simulink model "BLDC_180deg_realVSI"  (R2024a)
settings: Solver=ode15s  StartTime=0.0  StopTime=2  RelTol=1e-3
values from neighbouring files (symbols this model uses):
  D_m = 1e-3    (= 0.001)    [BLDC_Parameters.m]
  J_t = 1e-3    (= 0.001)    [BLDC_Parameters.m]
  L_ss = tau_s * r_s    (= 0.0003657)    [BLDC_Parameters.m]
  lambda_m = torque_const/(3*P/4)    (= 0.00985)    [BLDC_Parameters.m]
  P = 8    [BLDC_Parameters.m]
  r_s = r_pp/2    (= 0.345)    [BLDC_Parameters.m]
  R_vs = 1e6    (= 1000000)    [BLDC_Parameters.m]
  tau_s = 1.06e-3    (= 0.00106)    [BLDC_Parameters.m]
  V_bus = 12    [BLDC_Parameters.m]
libraries: simulink x7, spsMosfetLib x6, spsSeriesRLCBranchLib x4, spsVoltageMeasurementLib x3, spsControlledCurrentSourceLib x3, dspswit3 x1, slpidlib x1, spsPWMGeneratorDCDCLib x1, spsDCVoltageSourceLib x1, sps_lib x1
settings Model: Creator=matthewhasman  LastModifiedBy=matthewhasman

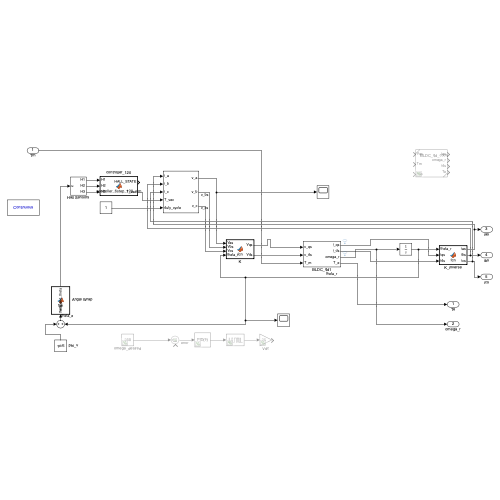
[thumbnail: Simulink's stored preview of the top-level diagram]
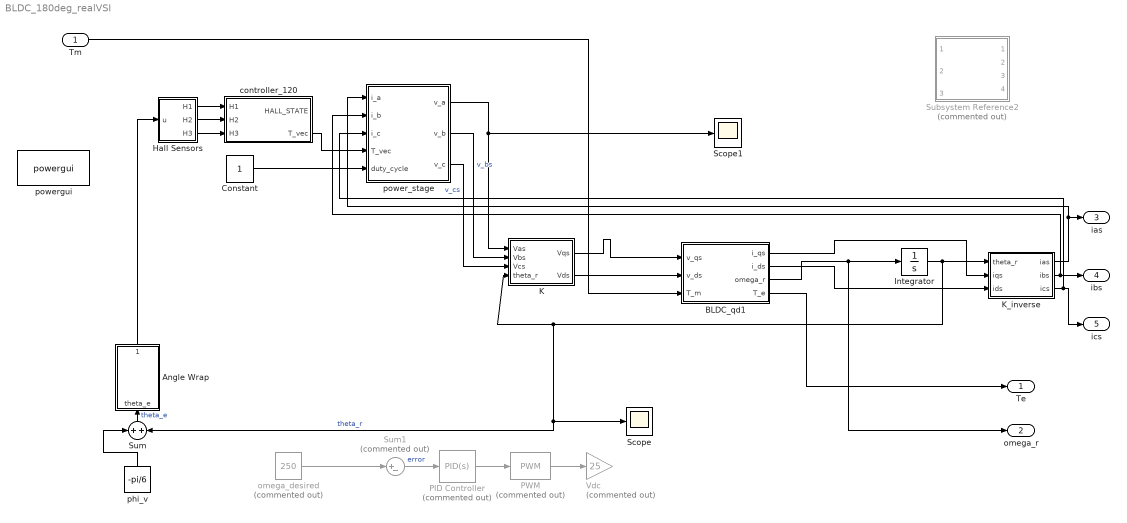
== system BLDC_180deg_realVSI ==
  Tm : Inport
  Angle Wrap : MATLAB Function  TreatAsAtomicUnit=on
  BLDC_qd1 : Subsystem
  Constant : Constant
  Hall Sensors : Subsystem
  Integrator : Integrator
  K : MATLAB Function  TreatAsAtomicUnit=on
  K_inverse : MATLAB Function  TreatAsAtomicUnit=on
  PID Controller : slpidlib/PID Controller  Commented=on  Controller=PID  Form=Parallel  TimeDomain=Continuous-time  UseExternalTs=off  SampleTime=-1  IntegratorMethod=Forward Euler  FilterMethod=Forward Euler  ControllerParametersSource=internal  P=8  I=5  UseKiTs=off  D=1  UseExternalDerivativeSource=off  N=100  UseFilter=on  TunerSelectOption=Transfer Function Based (PID Tuner App)  InitialConditionSource=internal  InitialConditionForIntegrator=0  InitialConditionForFilter=0  DifferentiatorICPrevScaledInput=0  ExternalReset=none  TrackingMode=off  Kt=1  LimitOutput=off  SatLimitsSource=internal  UpperSaturationLimit=inf  LowerSaturationLimit=-inf  LinearizeAsGain=on  AntiWindupMode=none  Kb=1  LimitIntegrator=off  UpperIntegratorSaturationLimit=inf  LowerIntegratorSaturationLimit=-inf  POutMin=[]  POutMax=[]  IOutMin=[]  IOutMax=[]  DOutMin=[]  DOutMax=[]  NOutMin=[]  NOutMax=[]  SumOutMin=[]  SumOutMax=[]  SaturationOutMin=[]  SaturationOutMax=[]  PParamMin=[]  PParamMax=[]  IParamMin=[]  IParamMax=[]  DParamMin=[]  DParamMax=[]  NParamMin=[]  NParamMax=[]  KbParamMin=[]  KbParamMax=[]  KtParamMin=[]  KtParamMax=[]  KbOutMin=[]  KbOutMax=[]  KtOutMin=[]  KtOutMax=[]  IntegratorOutMin=[]  IntegratorOutMax=[]  FilterOutMin=[]  FilterOutMax=[]  SumI1OutMin=[]  SumI1OutMax=[]  SumI2OutMin=[]  SumI2OutMax=[]  SumI3OutMin=[]  SumI3OutMax=[]  SumI4OutMin=[]  SumI4OutMax=[]  SumDOutMin=[]  SumDOutMax=[]  DifferentiatorOutMin=[]  DifferentiatorOutMax=[]  FilterDiffOutCoefMin=[]  FilterDiffOutCoefMax=[]  ReciprocalOutMin=[]  ReciprocalOutMax=[]  SumDenOutMin=[]  SumDenOutMax=[]  SumNumOutMin=[]  SumNumOutMax=[]  DivideOutMin=[]  DivideOutMax=[]  UdiffTsProdOutMin=[]  UdiffTsProdOutMax=[]  NTsProdOutMin=[]  NTsProdOutMax=[]  UintegralTsProdOutMin=[]  UintegralTsProdOutMax=[]  UngainTsProdOutMin=[]  UngainTsProdOutMax=[]  ClampingZeroOutDataTypeStr=Inherit: Inherit via back propagation  ClampingZeroOutMin=[]  ClampingZeroOutMax=[]  FilterDenConstantOutDataTypeStr=Inherit: Inherit via back propagation  FilterDenConstantOutMin=[]  FilterDenConstantOutMax=[]  PCopyOutDataTypeStr=Inherit: Inherit via back propagation  PCopyOutMin=[]  PCopyOutMax=[]  NCopyOutDataTypeStr=Inherit: Inherit via back propagation  NCopyOutMin=[]  NCopyOutMax=[]  IntegratorContinuousStateAttributes=''  IntegratorStateMustResolveToSignalObject=off  IntegratorRTWStateStorageClass=Auto  FilterContinuousStateAttributes=''  FilterStateMustResolveToSignalObject=off  FilterRTWStateStorageClass=Auto  ParallelPVariant=InternalParameters  IdealPVariant=Disabled  IVariant=InternalParameters  DVariant=InternalParameters  IntegratorVariant=Continuous  SatVariant=Disabled  AWVariant=Passthrough  PCopyVariant=Disabled  TRVariant=Disabled  FdbkBlocksVariant=Forward  IdealPFdbkVariant=Disabled  SatFdbkVariant=Disabled  DerivativeFilterVariant=ContFilter  NVariant=InternalParameters  NCopyVariant=Disabled  FilterICVariant=InternalICsFilter  IntegratorICVariant=InternalICs  ExternalResetVariant=Disabled  TRSumVariant=Passthrough  SumFdbkVariant=Disabled  SumVariant=Sum_PID  TsampFilterVariant=InternalTs  TsampNgainVariant=Passthrough  TsampIntegralVariant=Disabled_SignalSpec  ExternalSaturationOutDataTypeStr=Inherit: Same as second input  DerivativeSourceVariant=ErrorSignal
  PWM : simulink/Discontinuities/PWM  Commented=on  DisableCoverage=on  Period=0.0001  InitialDelay=0  DisallowZeroDutyCycle=off  RunAtFixedTimeIntervals=off  SampleTime=0.1
  Scope : Scope
  Scope1 : Scope
  Subsystem Reference2 : Subsystem  Commented=on  ReferencedSubsystem=BLDC_qd_coords
  Sum : Sum
  Sum1 : Sum  Commented=on  Inputs=|+-
  Vdc : Gain  Commented=on  Gain=25
  controller_120 : MATLAB Function  TreatAsAtomicUnit=on
  omega_desired : Constant  Commented=on  Value=250
  phi_v : Constant  Value=-pi/6
  power_stage : Subsystem
  powergui : sps_lib/powergui  Priority=1  SimulationMode=Continuous  SampleTime=50e-6  frequency=60  Iterations=50  frequencyindice=0  Pbase=100e6  ErrMax=1e-4  UnitsV=kV  UnitsW=MW  buscounter=0  FunctionMessages=off  echomessages=off  EnableUseOfTLC=off  CurrentSourceSwitches=off  DisableSnubberDevices=off  DisableRonSwitches=off  DisableVfSwitches=off  DisplayEquations=off  AutomaticDiscreteSolvers=off  SolverType=Tustin/Backward Euler (TBE)  Interpol=off  ExternalGateDelay=off  methode=off  Ts=100  x0status=blocks  SPID=on  SwTol=0  HookPort=off  NonlinearTolerance=1e-4  nMaxIteration=100  ContinueOnMaxIteration=off  RestoreLinks=warning  ResistiveCurrentMeasurement=off  Frange=[0:2:500]  Ylog=off  Xlog=on  ShowGrid=off  save=off  variable=ZData  structure=0  ZoomFFT=off  StartTime=0.0  cycles=1  DisplayStyle=1  fundamental=60  FreqAxis=off  MaxFrequency=1000  frequencyindicesteady=1  RmsSteady=1  display=off
  Te : Outport
  omega_r : Outport  Port=2
  ias : Outport  Port=3
  ibs : Outport  Port=4
  ics : Outport  Port=5
  wires:
  Integrator/1 -> K_inverse/1(theta_r), Scope/1, Sum/2, K/4(theta_r)  "theta_r"
  K/1(Vqs) -> BLDC_qd1/1(v_qs)
  phi_v/1 -> Sum/1
  power_stage/1(v_a) -> Scope1/1, K/1(Vas)
  omega_desired/1 -> Sum1/1
  Sum1/1 -> PID Controller/1  "error"
  PID Controller/1 -> PWM/1
  PWM/1 -> Vdc/1
  Sum/1 -> Angle Wrap/1(theta_e)  "theta_e"
  K_inverse/1(ias) -> power_stage/1(i_a), ias/1
  K_inverse/2(ibs) -> ibs/1, power_stage/2(i_b)
  K_inverse/3(ics) -> power_stage/3(i_c), ics/1
  Angle Wrap/1(wrapped_theta) -> Hall Sensors/1(u)
  power_stage/2(v_b) -> K/2(Vbs)  "v_bs"
  power_stage/3(v_c) -> K/3(Vcs)  "v_cs"
  Hall Sensors/3(H3) -> controller_120/3(H3)
  Hall Sensors/1(H1) -> controller_120/1(H1)
  Hall Sensors/2(H2) -> controller_120/2(H2)
  controller_120/2(T_vec) -> power_stage/4(T_vec)
  Constant/1 -> power_stage/5(duty_cycle)
  K/2(Vds) -> BLDC_qd1/2(v_ds)
  Tm/1 -> BLDC_qd1/3(T_m)
  BLDC_qd1/1(i_qs) -> K_inverse/2(iqs)
  BLDC_qd1/2(i_ds) -> K_inverse/3(ids)
  BLDC_qd1/3(omega_r) -> omega_r/1, Integrator/1
  BLDC_qd1/4(T_e) -> Te/1

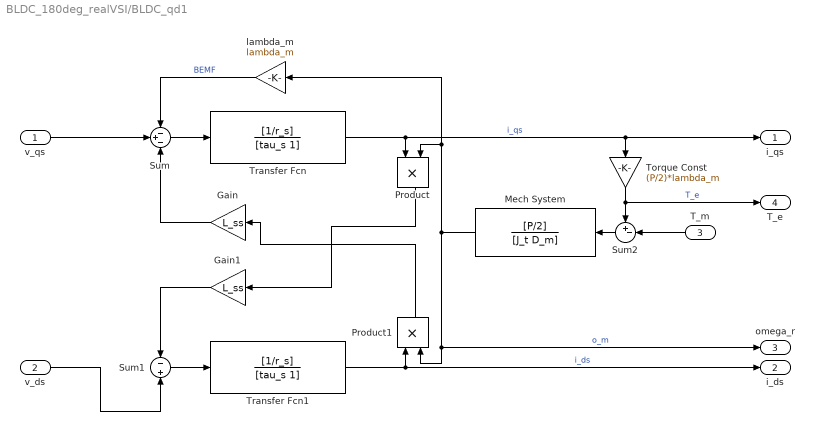
== system BLDC_180deg_realVSI/BLDC_qd1 ==
  v_qs : Inport
  v_ds : Inport  Port=2
  T_m : Inport  Port=3
  Gain : Gain  Gain=L_ss
  Gain1 : Gain  Gain=L_ss
  Mech System : TransferFcn  Numerator=[P/2]  Denominator=[J_t D_m]
  Product : Product
  Product1 : Product
  Sum : Sum  Inputs=-+-
  Sum1 : Sum  Inputs=-+
  Sum2 : Sum  Inputs=+-|
  Torque Const : Gain  Gain=(P/2)*lambda_m
  Transfer Fcn : TransferFcn  Numerator=[1/r_s]  Denominator=[tau_s 1]
  Transfer Fcn1 : TransferFcn  Numerator=[1/r_s]  Denominator=[tau_s 1]
  lambda_m : Gain  Gain=lambda_m
  i_qs : Outport
  i_ds : Outport  Port=2
  omega_r : Outport  Port=3
  T_e : Outport  Port=4
  wires:
  T_m/1 -> Sum2/2
  Sum1/1 -> Transfer Fcn1/1
  Gain1/1 -> Sum1/1
  Product1/1 -> Gain/1
  Transfer Fcn1/1 -> i_ds/1, Product1/1  "i_ds"
  Mech System/1 -> lambda_m/1, Product/2, omega_r/1, Product1/2  "o_m"
  Torque Const/1 -> T_e/1, Sum2/1  "T_e"
  v_ds/1 -> Sum1/2
  Transfer Fcn/1 -> i_qs/1, Torque Const/1, Product/1  "i_qs"
  Product/1 -> Gain1/1
  Gain/1 -> Sum/3
  v_qs/1 -> Sum/2
  Sum/1 -> Transfer Fcn/1
  Sum2/1 -> Mech System/1
  lambda_m/1 -> Sum/1  "BEMF"

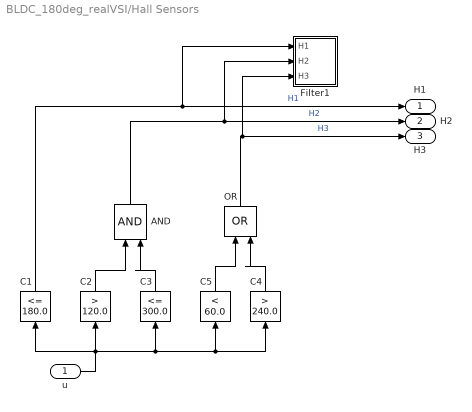
== system BLDC_180deg_realVSI/Hall Sensors ==
  u : Inport
  AND : Logic  IconShape=distinctive  AllPortsSameDT=off  OutDataTypeStr=boolean
  C1 : simulink/Logic and Bit Operations/Compare To Constant  relop=<=  const=180.0  OutDataTypeStr=boolean
  C2 : simulink/Logic and Bit Operations/Compare To Constant  relop=>  const=120.0  OutDataTypeStr=boolean
  C3 : simulink/Logic and Bit Operations/Compare To Constant  relop=<=  const=300.0  OutDataTypeStr=boolean
  C4 : simulink/Logic and Bit Operations/Compare To Constant  relop=>  const=240.0  OutDataTypeStr=boolean
  C5 : simulink/Logic and Bit Operations/Compare To Constant  relop=<  const=60.0  OutDataTypeStr=boolean
  Filter1 : Subsystem
  OR : Logic  Operator=OR  IconShape=distinctive  AllPortsSameDT=off  OutDataTypeStr=boolean
  H1 : Outport
  H2 : Outport  Port=2
  H3 : Outport  Port=3
  wires:
  C4/1 -> OR/2
  C1/1 -> H1/1, Filter1/1(H1)  "H1"
  OR/1 -> H3/1, Filter1/3(H3)  "H3"
  C3/1 -> AND/2
  AND/1 -> H2/1, Filter1/2(H2)  "H2"
  u/1 -> C2/1, C5/1, C4/1, C3/1, C1/1
  C2/1 -> AND/1
  C5/1 -> OR/1

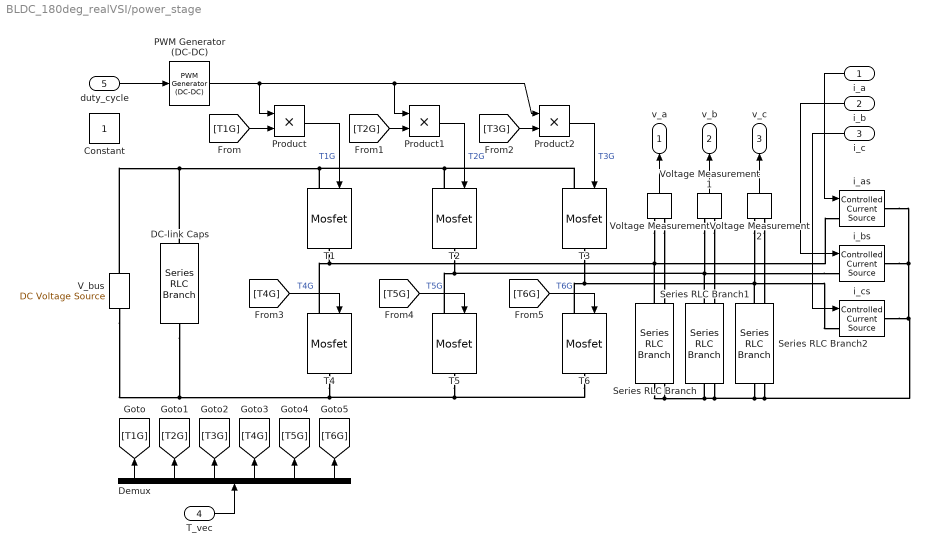
== system BLDC_180deg_realVSI/power_stage ==
  i_a : Inport
  i_b : Inport  Port=2
  i_c : Inport  Port=3
  T_vec : Inport  Port=4
  duty_cycle : Inport  Port=5
  Constant : Constant
  DC-link Caps : spsSeriesRLCBranchLib/Series RLC Branch  LConnTagsString=__new0  RConnTagsString=__new0  BranchType=RC  Resistance=1e-6  Inductance=0  SetiL0=off  InitialCurrent=0  Capacitance=100e-6  Setx0=off  InitialVoltage=0  Measurements=None
  Demux : Demux  Outputs=6
  PWM Generator (DC-DC) : spsPWMGeneratorDCDCLib/PWM Generator (DC-DC)  Fsw=f_SW_Hz  Ts=0
  Product : Product
  Product1 : Product
  Product2 : Product
  Series RLC Branch : spsSeriesRLCBranchLib/Series RLC Branch  LConnTagsString=__new0  RConnTagsString=__new0  BranchType=R  Resistance=R_vs  Inductance=0  SetiL0=off  InitialCurrent=0  Capacitance=inf  Setx0=off  InitialVoltage=0  Measurements=None
  Series RLC Branch1 : spsSeriesRLCBranchLib/Series RLC Branch  LConnTagsString=__new0  RConnTagsString=__new0  BranchType=R  Resistance=R_vs  Inductance=0  SetiL0=off  InitialCurrent=0  Capacitance=inf  Setx0=off  InitialVoltage=0  Measurements=None
  Series RLC Branch2 : spsSeriesRLCBranchLib/Series RLC Branch  LConnTagsString=__new0  RConnTagsString=__new0  BranchType=R  Resistance=R_vs  Inductance=0  SetiL0=off  InitialCurrent=0  Capacitance=inf  Setx0=off  InitialVoltage=0  Measurements=None
  T{1..6} (6 alike) : spsMosfetLib/Mosfet  Ron=R_dsON_Ohm  Lon=0  Rd=0.01  Vfd=0.7  IC=0  Rs=1e5  Cs=inf  Measurements=off
  V_bus : spsDCVoltageSourceLib/DC Voltage Source  Amplitude=V_bus  Measurements=None
  Voltage Measurement : spsVoltageMeasurementLib/Voltage Measurement  PhasorSimulation=off  OutputType=Complex  PSBequivalent=0
  Voltage Measurement1 : spsVoltageMeasurementLib/Voltage Measurement  PhasorSimulation=off  OutputType=Complex  PSBequivalent=0
  Voltage Measurement2 : spsVoltageMeasurementLib/Voltage Measurement  PhasorSimulation=off  OutputType=Complex  PSBequivalent=0
  i_as : spsControlledCurrentSourceLib/Controlled Current Source  Initialize=on  Source_Type=AC  Amplitude=0  Phase=0  Frequency=0  Measurements=None
  i_bs : spsControlledCurrentSourceLib/Controlled Current Source  Initialize=on  Source_Type=AC  Amplitude=0  Phase=0  Frequency=0  Measurements=None
  i_cs : spsControlledCurrentSourceLib/Controlled Current Source  Initialize=on  Source_Type=AC  Amplitude=0  Phase=0  Frequency=0  Measurements=None
  v_a : Outport
  v_b : Outport  Port=2
  v_c : Outport  Port=3
  wires:
  T_vec/1 -> Demux/1
  Product1/1 -> T2/1  "T2G"
  PWM Generator (DC-DC)/1 -> Product/1, Product2/1, Product1/1
  Demux/6 -> [T6G]
  [T4G] -> T4/1  "T4G"
  [T5G] -> T5/1  "T5G"
  Demux/4 -> [T4G]
  Voltage Measurement/1 -> v_a/1
  [T2G] -> Product1/2
  Voltage Measurement1/1 -> v_b/1
  Voltage Measurement2/1 -> v_c/1
  i_a/1 -> i_as/1
  Demux/1 -> [T1G]
  Demux/5 -> [T5G]
  [T6G] -> T6/1  "T6G"
  i_c/1 -> i_cs/1
  Product/1 -> T1/1  "T1G"
  [T3G] -> Product2/2
  i_b/1 -> i_bs/1
  Product2/1 -> T3/1  "T3G"
  Demux/2 -> [T2G]
  Demux/3 -> [T3G]
  [T1G] -> Product/2
  duty_cycle/1 -> PWM Generator (DC-DC)/1
  connections:
  i_bs/LConn1 -- Voltage Measurement1/LConn1 -- Series RLC Branch1/LConn1 -- T2/RConn1 -- T5/LConn1
  DC-link Caps/RConn1 -- V_bus/LConn1 -- T4/RConn1 -- T6/RConn1 -- T5/RConn1
  DC-link Caps/LConn1 -- V_bus/RConn1 -- T1/LConn1 -- T3/LConn1 -- T2/LConn1
  T4/LConn1 -- T1/RConn1 -- Voltage Measurement/LConn1 -- Series RLC Branch/LConn1 -- i_as/LConn1
  T3/RConn1 -- T6/LConn1 -- Voltage Measurement2/LConn1 -- Series RLC Branch2/LConn1 -- i_cs/LConn1
  Series RLC Branch/RConn1 -- Voltage Measurement/LConn2 -- i_bs/RConn1 -- i_as/RConn1 -- i_cs/RConn1 -- Voltage Measurement2/LConn2 -- Series RLC Branch2/RConn1 -- Voltage Measurement1/LConn2 -- Series RLC Branch1/RConn1

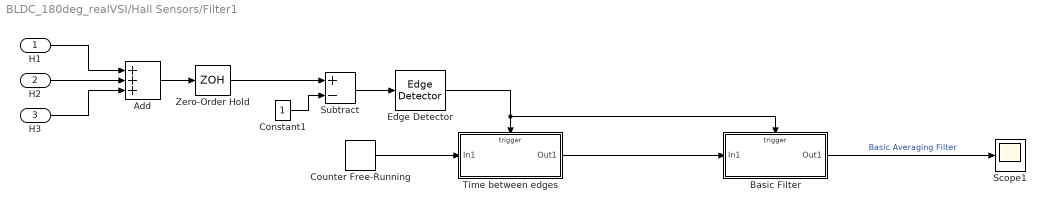
== system BLDC_180deg_realVSI/Hall Sensors/Filter1 ==
  H1 : Inport
  H2 : Inport  Port=2
  H3 : Inport  Port=3
  Add : Sum  Inputs=+++
  Basic Filter : Subsystem  TreatAsAtomicUnit=on
  Constant1 : Constant
  Counter Free-Running : simulink/Sources/Counter Free-Running  NumBits=16  tsamp=0.0001
  Edge Detector : dspswit3/Edge Detector  InputProcessing=Columns as channels (frame based)
  Scope1 : Scope
  Subtract : Sum  Inputs=+-
  Time between edges : Subsystem  TreatAsAtomicUnit=on
  Zero-Order Hold : ZeroOrderHold  SampleTime=0.0001
  wires:
  H3/1 -> Add/3
  Counter Free-Running/1 -> Time between edges/1(In1)
  H1/1 -> Add/1
  Constant1/1 -> Subtract/2
  Add/1 -> Zero-Order Hold/1
  Edge Detector/1 -> Basic Filter/Trigger, Time between edges/Trigger
  Subtract/1 -> Edge Detector/1
  H2/1 -> Add/2
  Zero-Order Hold/1 -> Subtract/1
  Time between edges/1(Out1) -> Basic Filter/1(In1)
  Basic Filter/1(Out1) -> Scope1/1  "Basic Averaging Filter"

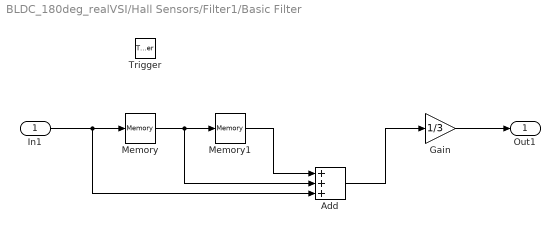
== system BLDC_180deg_realVSI/Hall Sensors/Filter1/Basic Filter ==
  In1 : Inport
  Trigger : TriggerPort  VariantControl=(inherit)
  Add : Sum  Inputs=+++
  Gain : Gain  Gain=1/3
  Memory : Memory  InheritSampleTime=on
  Memory1 : Memory  InheritSampleTime=on
  Out1 : Outport
  wires:
  In1/1 -> Add/3, Memory/1
  Memory/1 -> Add/2, Memory1/1
  Memory1/1 -> Add/1
  Add/1 -> Gain/1
  Gain/1 -> Out1/1

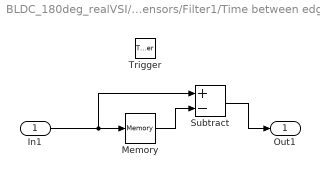
== system BLDC_180deg_realVSI/Hall Sensors/Filter1/Time between edges ==
  In1 : Inport
  Trigger : TriggerPort  VariantControl=(inherit)
  Memory : Memory  InheritSampleTime=on
  Subtract : Sum  Inputs=+-
  Out1 : Outport
  wires:
  In1/1 -> Subtract/1, Memory/1
  Memory/1 -> Subtract/2
  Subtract/1 -> Out1/1

== matlab function BLDC_180deg_realVSI/K ==
  data: Vas input; Vqs output; Vbs input; Vcs input; Vds output; theta_r input
function [Vqs, Vds] = fcn(Vas, Vbs, Vcs, theta_r)
offset = 2*pi/3;
k = (2/3)*[cos(theta_r), cos(theta_r - offset), cos(theta_r + offset);
           sin(theta_r), sin(theta_r - offset), sin(theta_r + offset)];

qds_voltage = k * [Vas; Vbs; Vcs];

Vqs = qds_voltage(1);
Vds = qds_voltage(2);

end

== matlab function BLDC_180deg_realVSI/K_inverse ==
  data: theta_r input; ias output; iqs input; ids input; ibs output; ics output
function [ias, ibs, ics] = fcn(theta_r, iqs, ids)
offset = 2*pi/3;
k_inverse = [cos(theta_r), sin(theta_r);
             cos(theta_r - offset), sin(theta_r - offset);
             cos(theta_r + offset), sin(theta_r + offset)];

abc_currents = k_inverse * [iqs; ids];

ias = abc_currents(1);
ibs = abc_currents(2);
ics = abc_currents(3);

end

== matlab function BLDC_180deg_realVSI/Angle Wrap ==
  data: theta_e input; wrapped_theta output
function wrapped_theta = fcn(theta_e)

wrapped_theta = wrapTo2Pi(theta_e) * 180 / pi;

== matlab function BLDC_180deg_realVSI/controller_120 ==
  data: H1 input; HALL_STATE output; H2 input; H3 input; T_vec output
function [HALL_STATE, T_vec] = controller_6step_120_sim(H1,H2,H3)
[HALL_STATE, T_vec] = controller_6step_120(H1,H2,H3);
end
